simulink model "es6_sim_rumore"  (Simulink 7.9)
settings: Solver=ode45  StartTime=0.0  StopTime=10  RelTol=1e-3
values from neighbouring files (symbols this model uses):
  A = [-7 -12;-1 -3]    [es6.m]    (also in es6b.m)
  B = [1 1]'    [es6.m]    (also in es6b.m)
  C = [1 1]    [es6.m]    (also in es6b.m)
  L = place(A',C',10*E)'    [es6.m]
  X0 = [1 1]    [es6.m]
  X0obsv = [0 0]    [es6.m]
undefined symbols (not defined in the file or in its folder): K, sigbuilder_block
settings Model: Creator=claudio  LastModifiedBy=patrizio
settings OptimizationCC: InlineInvariantSignals=on  InitFltsAndDblsToZero=on
settings DebuggingCC: SaveWithParameterizedLinksMsg=none  SignalResolutionControl=TryResolveAllWithWarning  MultiTaskDSMMsg=warning  MultiTaskCondExecSysMsg=none  FcnCallInpInsideContextMsg=Use local settings  StrictBusMsg=None
settings RTWCC: IncludeERTFirstTime=on
settings GRTTargetCC: TargetFcnLib=ansi_tfl_tmw.mat  CombineOutputUpdateFcns=off  GRTInterface=on

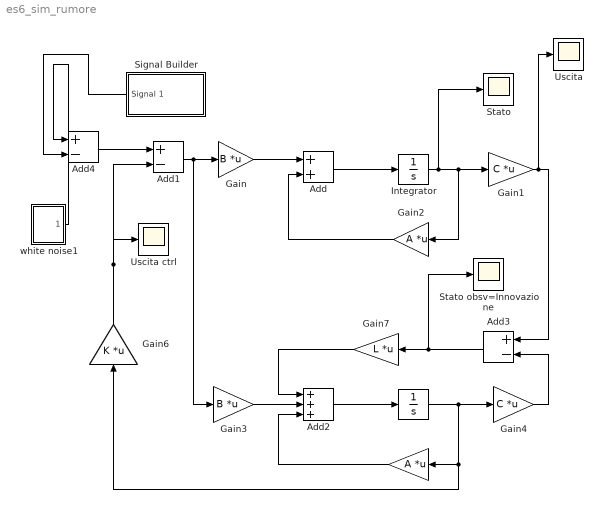
== system es6_sim_rumore ==
  " " : Integrator  InitialCondition=X0obsv
  "   " : Gain  Gain=A  Multiplication=Matrix(K*u)
  Add : Sum
  Add1 : Sum  Inputs=+-
  Add2 : Sum  Inputs=+++
  Add3 : Sum  Inputs=+-
  Add4 : Sum  Inputs=+-
  Gain : Gain  Gain=B  Multiplication=Matrix(K*u)
  Gain1 : Gain  Gain=C  Multiplication=Matrix(K*u)
  Gain2 : Gain  Gain=A  Multiplication=Matrix(K*u)
  Gain3 : Gain  Gain=B  Multiplication=Matrix(K*u)
  Gain4 : Gain  Gain=C  Multiplication=Matrix(K*u)
  Gain6 : Gain  Gain=K  Multiplication=Matrix(K*u)
  Gain7 : Gain  Gain=L  Multiplication=Matrix(K*u)
  Integrator : Integrator  InitialCondition=X0
  Signal Builder : Subsystem  Tag=STV Subsys  LoadFcn=sigbuilder_block('load');  StartFcn=sigbuilder_block('start');  StopFcn=sigbuilder_block('stop');  ClipboardFcn=sigbuilder_block('clipboard');  mask(Sigbuilder block){}
      mask help: Sigbuilder GUI
      mask init:
      | if ~strcmp(get_param(bdroot(gcbh),'SimulationStatus'),'stopped') tuvar = sigbuilder_block('maskInit'); end
      settings: CopyFcn=sigbuilder_block('copy');  DeleteFcn=sigbuilder_block('delete');  ModelCloseFcn=sigbuilder_block('modelClose');  PreSaveFcn=sigbuilder_block('preSave');  PauseFcn=sigbuilder_block('pause')  ContinueFcn=sigbuilder_block('continue')  NameChangeFcn=sigbuilder_block('namechange');  OpenFcn=sigbuilder_block('open',[488 73.6 520 400 ]);  CloseFcn=sigbuilder_block('close');
      mask Display: plot(0,0,100,100,[10,10,40,40,10],[80,20,20,80,80],[40,10],[50,50], [40,27,10],[65,72,56],[40,25,25,10],[28,28,43,43]);
  Stato : Scope
      settings: SaveName=ScopeData3
  Stato obsv=Innovazione : Scope
  Uscita : Scope
      settings: TimeRange=10  SaveName=ScopeData2
  Uscita ctrl : Scope
  white noise1 : Subsystem  mask(Continuous White Noise.){Cov=1, Ts=0.1, seed=12}
      mask prompts: Cov "Noise Variance:"; Ts "Sample Time:"
      mask help:
      | White noise for continuous (s-domain) systems.
      | Band-limited using zero-order-hold.
      mask Help: Implemented using white noise into Zero Order Hold block. For faster simulation set sample time to highest value possible but in accordance with the fastest dynamics of system.
      mask Display: plot(1:20,rand(1,20))
  wires:
  Integrator/1 -> Gain1/1, Gain2/1, Stato/1
  Add/1 -> Integrator/1
  Gain2/1 -> Add/2
  Gain/1 -> Add/1
  Add1/1 -> Gain/1, Gain3/1
  " "/1 -> Gain4/1, "   "/1, Gain6/1
  Add2/1 -> " "/1
  Gain6/1 -> Uscita ctrl/1, Add1/2
  Gain4/1 -> Add3/2
  Gain1/1 -> Add3/1, Uscita/1
  Add3/1 -> Gain7/1, Stato obsv=Innovazione/1
  Gain7/1 -> Add2/1
  Gain3/1 -> Add2/2
  "   "/1 -> Add2/3
  white noise1/1(out_1) -> Add4/1
  Add4/1 -> Add1/1
  Signal Builder/1(Signal 1) -> Add4/2

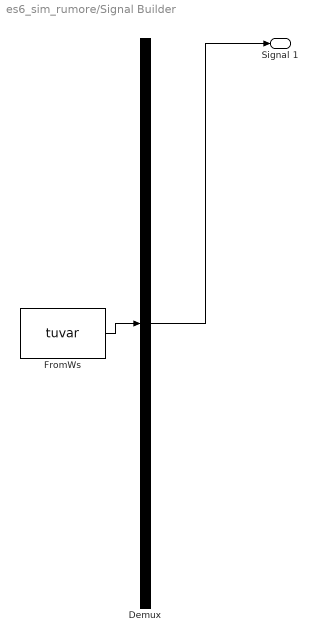
== system es6_sim_rumore/Signal Builder ==
  Demux : Demux  Tag=STV Demux  Outputs=1
  FromWs : FromWorkspace  Tag=STV FromWs  VariableName=tuvar  SampleTime=0  SigBuilderData=DataTag0  VnvData=DataTag1
      SigBuilderData=|
      | dataSet.timeRange = [0 10]
      | dataSet.name = 'Group 1'
      | sbobj.Name = 'Signal Builder'
      | sbobj.Groups.Name = 'Group 1'
      | sbobj.Groups.Signals.Name = 'Signal 1'
      | sbobj.Groups.Signals.XData = [0 1 5 5 6 6 10]
      | sbobj.Groups.Signals.YData = [0 0 0 5 5 0 0]
  Signal 1 : Outport  Tag=STV Outport
  wires:
  Demux/1 -> Signal 1/1
  FromWs/1 -> Demux/1

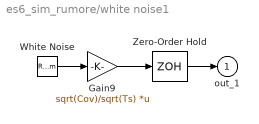
== system es6_sim_rumore/white noise1 ==
  Gain9 : Gain  Gain=sqrt(Cov)/sqrt(Ts)  Multiplication=Matrix(K*u)
  White Noise : RandomNumber  Mean=zeros(length(Cov),1)  Variance=ones(length(Cov),1)  Seed=seed
  Zero-Order Hold : ZeroOrderHold  SampleTime=Ts
  out_1 : Outport
  wires:
  Gain9/1 -> Zero-Order Hold/1
  White Noise/1 -> Gain9/1
  Zero-Order Hold/1 -> out_1/1
